simulink model "Trabajo3_linealizacion"  (R2024b)
settings: Solver=ode45  StartTime=0.0  StopTime=30  MaxStep=0.01  RelTol=1e-3  EnableMultiTasking=on
undefined symbols (not defined in the file): Beta, c, CI, f, g, l, m, Mu, Ts, V
settings Model: Creator=CarlosM  LastModifiedBy=Juanj
settings SolverCC: AlgebraicLoopSolver=TrustRegion
settings DataIOCC: SaveFormat=Array  SaveOutput=off  SignalLogging=off  DSMLogging=off  SaveTime=off  ReturnWorkspaceOutputs=off
settings OptimizationCC: ReuseModelBlockBuffer=off  LifeSpan=inf
settings DebuggingCC: UnderspecifiedInitializationDetection=Classic  MergeDetectMultiDrivingBlocksExec=none  SolverPrmCheckMsg=warning  UnconnectedInputMsg=warning  UnconnectedOutputMsg=warning  UnconnectedLineMsg=warning  StateNameClashWarn=warning  SFUnexpectedBacktrackingDiag=warning  SFNoUnconditionalDefaultTransitionDiag=warning  SFExecutionAtInitializationDiag=none  ArithmeticOperatorsInVariantConditions=warning
settings HardwareCC: ProdBitPerPointer=32  ProdBitPerSizeT=32  ProdBitPerPtrDiffT=32  ProdLargestAtomicFloat=None  ProdIntDivRoundTo=Undefined  ProdEndianess=Unspecified  ProdWordSize=32  ProdHWDeviceType=32-bit Generic
settings ModelReferenceCC: EnableRefExpFcnMdlSchedulingChecks=on  PropagateSignalLabelsOutOfModel=off
settings SFSimCC: SimUseLocalCustomCode=off  CustomCodeUndefinedFunction=UseInterfaceOnly
settings RTWCC: RTWUseLocalCustomCode=off  GPUComputeCapability=3.5  DLArmComputeVersion=19.05
settings CodeAppCC: StateflowObjectComments=on
settings GRTTargetCC: TargetLangStandard=C89/C90 (ANSI)
settings ConfigComp: CovMetricSettings=dw  CovSaveCumulativeToWorkspaceVar=on  CovSaveSingleToWorkspaceVar=on  CovExternalEMLEnable=off

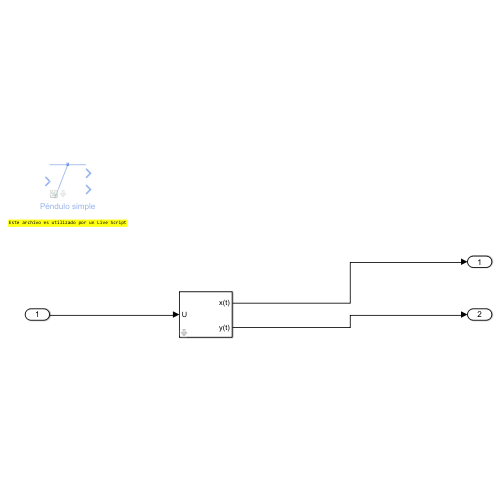
[thumbnail: Simulink's stored preview of the top-level diagram]
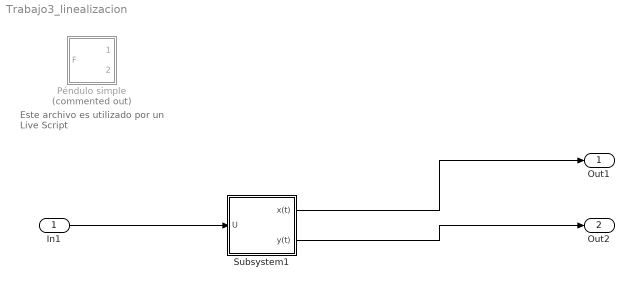
== system Trabajo3_linealizacion ==
  note: Este archivo es utilizado por un Live Script
  In1 : Inport
  Péndulo simple : Subsystem  Commented=on  mask(Modelo de un péndulo simple con una fuerza tangencial){par=[m l g f], x0=[0 0], noise=off}
      mask prompts: par "[m l g f]"; x0 "Condiciones iniciales (th0, omega0)"; noise "Incluir ruido"
      mask help:
      | Modelo no lineal
      | Entrada: fuerza externa tangencial al movimiento (u = F)
      | Salidas: posición angular (x1  = theta), velocidad angular (x2 = omega = theta')
      mask init:
      | m=par(1); l=par(2); g=par(3); f=par(4);
      mask Help:
      | Ecuación de estado:
      | x1' = x2
      | x2' = -(g/l)*sen(x1) - (f/m)*x2 + u/(m*l)
      | 
      | Parámetros:
      | m - Masa
      | l - Longitud del péndulo
      | g - Aceleración de la gravedad
      | f - Coeficiente de fricción viscosa
      mask Display: plot([.1,.9],[.9,.9],[.5,.2],[.9,.25],[.475,.475,.525,.525,.475],[.875,.925,.925,.875,.875])
  Subsystem1 : Subsystem  mask{Beta=Beta, Mu=Mu, V=V, c=c, X0=CI}
      mask prompts: Beta "Tasa de Transmisión (Beta)"; Mu "Tasa de Muertes (Mu)"; V "Tasa de Recuperación (V)"; c "Contactos Suceptibles-Infectados (c)"; X0 "Suceptibles Iniciales (X0)"
  Out1 : Outport
  Out2 : Outport  Port=2
  wires:
  Subsystem1/1(x(t)) -> Out1/1
  Subsystem1/2(y(t)) -> Out2/1
  In1/1 -> Subsystem1/1(U)

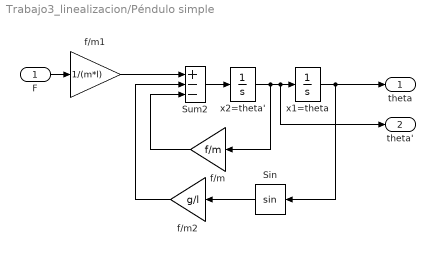
== system Trabajo3_linealizacion/Péndulo simple ==
  F : Inport
  Sin : Trigonometry
  Sum2 : Sum  Inputs=+--  InputSameDT=on  SaturateOnIntegerOverflow=on  OutDataTypeStr=Inherit: Same as first input
  f/m : Gain  Gain=f/m  SaturateOnIntegerOverflow=on  OutDataTypeStr=Inherit: Same as input  ParamDataTypeStr=Inherit: Same as input
  f/m1 : Gain  Gain=1/(m*l)  SaturateOnIntegerOverflow=on  OutDataTypeStr=Inherit: Same as input  ParamDataTypeStr=Inherit: Same as input
  f/m2 : Gain  Gain=g/l  SaturateOnIntegerOverflow=on  OutDataTypeStr=Inherit: Same as input  ParamDataTypeStr=Inherit: Same as input
  x1=theta : Integrator  InitialCondition=x0(1)
  x2=theta' : Integrator  InitialCondition=x0(2)
  theta : Outport
  theta' : Outport  Port=2
  wires:
  x1=theta/1 -> theta/1, Sin/1
  F/1 -> f/m1/1
  Sum2/1 -> x2=theta'/1
  x2=theta'/1 -> f/m/1, x1=theta/1, theta'/1
  f/m2/1 -> Sum2/2
  f/m/1 -> Sum2/3
  f/m1/1 -> Sum2/1
  Sin/1 -> f/m2/1

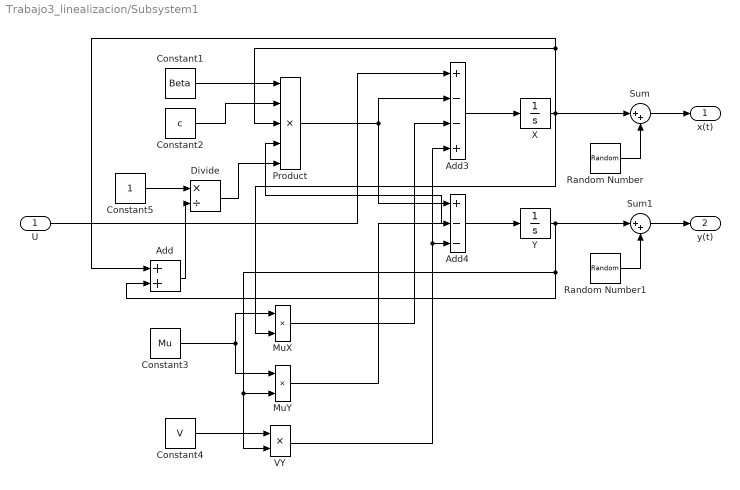
== system Trabajo3_linealizacion/Subsystem1 ==
  U : Inport
  Add : Sum
  Add3 : Sum  Inputs=+--+
  Add4 : Sum  Inputs=+--
  Constant1 : Constant  Value=Beta
  Constant2 : Constant  Value=c
  Constant3 : Constant  Value=Mu
  Constant4 : Constant  Value=V
  Constant5 : Constant
  Divide : Product  Inputs=*/
  MuX : Product
  MuY : Product
  Product : Product  Inputs=5
  Random Number : RandomNumber  Variance=64  SampleTime=Ts
  Random Number1 : RandomNumber  Variance=640  SampleTime=Ts
  Sum : Sum  Inputs=|++
  Sum1 : Sum  Inputs=|++
  VY : Product
  X : Integrator  InitialCondition=X0(1)  LimitOutput=on  LowerSaturationLimit=0
  Y : Integrator  InitialCondition=X0(2)  LimitOutput=on  LowerSaturationLimit=0
  x(t) : Outport
  y(t) : Outport  Port=2
  wires:
  X/1 -> Sum/1, Add/1, Product/3, MuX/2
  MuY/1 -> Add4/2
  Divide/1 -> Product/5
  Y/1 -> Sum1/1, Add/2, MuY/2, VY/2, Product/4
  Constant1/1 -> Product/1
  MuX/1 -> Add3/3
  Constant4/1 -> VY/1
  Add3/1 -> X/1
  Product/1 -> Add4/1, Add3/2
  Constant3/1 -> MuX/1, MuY/1
  U/1 -> Add3/1
  Add4/1 -> Y/1
  Constant2/1 -> Product/2
  Constant5/1 -> Divide/1
  VY/1 -> Add4/3, Add3/4
  Add/1 -> Divide/2
  Random Number/1 -> Sum/2
  Sum/1 -> x(t)/1
  Random Number1/1 -> Sum1/2
  Sum1/1 -> y(t)/1
